simulink library "adc"  (Simulink 8.1)
settings: Solver=ode45  StartTime=0.0  StopTime=10.0  RelTol=1e-3
undefined symbols (not defined in the file or in its folder): KJUD_AEBDeactVehSpeed_mps, KJUD_AEBVehAssignTimer_ms
libraries: ava x1, hcu_lib x1
settings Model: Creator=xsellart  LastModifiedBy=tescamilla

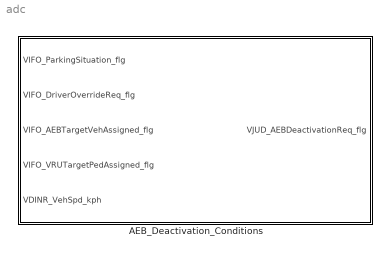
== system adc ==
  AEB_Deactivation_Conditions : Subsystem

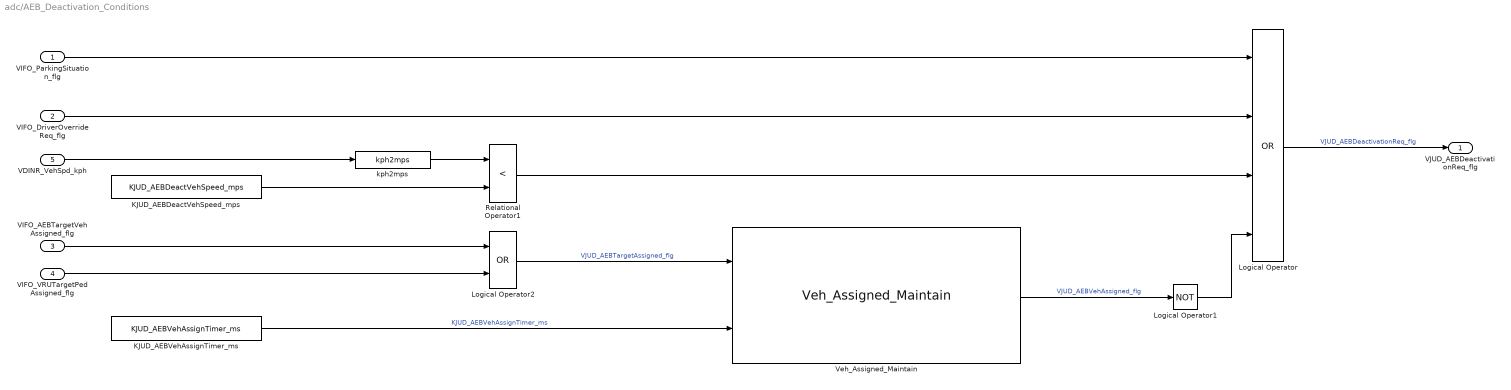
== system adc/AEB_Deactivation_Conditions ==
  VIFO_ParkingSituation_flg : Inport
  VIFO_DriverOverrideReq_flg : Inport  Port=2
  VIFO_AEBTargetVehAssigned_flg : Inport  Port=3
  VIFO_VRUTargetPedAssigned_flg : Inport  Port=4
  VDINR_VehSpd_kph : Inport  Port=5
  KJUD_AEBDeactVehSpeed_mps : Constant  Value=KJUD_AEBDeactVehSpeed_mps  OutDataTypeStr=single
  KJUD_AEBVehAssignTimer_ms : Constant  Value=KJUD_AEBVehAssignTimer_ms  OutDataTypeStr=single
  Logical Operator : Logic  Operator=OR  Inputs=4  AllPortsSameDT=off  OutDataTypeStr=boolean
  Logical Operator1 : Logic  Operator=NOT  AllPortsSameDT=off  OutDataTypeStr=boolean
  Logical Operator2 : Logic  Operator=OR  AllPortsSameDT=off  OutDataTypeStr=boolean
  Relational Operator1 : RelationalOperator  Operator=<  OutDataTypeStr=boolean
  Veh_Assigned_Maintain : ava/Veh_Assigned_Maintain
  kph2mps : hcu_lib/kph2mps
  VJUD_AEBDeactivationReq_flg : Outport
  wires:
  Logical Operator/1 -> VJUD_AEBDeactivationReq_flg/1  "VJUD_AEBDeactivationReq_flg"
  VIFO_AEBTargetVehAssigned_flg/1 -> Logical Operator2/1
  Relational Operator1/1 -> Logical Operator/3
  KJUD_AEBDeactVehSpeed_mps/1 -> Relational Operator1/2
  VDINR_VehSpd_kph/1 -> kph2mps/1
  VIFO_DriverOverrideReq_flg/1 -> Logical Operator/2
  VIFO_ParkingSituation_flg/1 -> Logical Operator/1
  Logical Operator1/1 -> Logical Operator/4
  KJUD_AEBVehAssignTimer_ms/1 -> Veh_Assigned_Maintain/2  "KJUD_AEBVehAssignTimer_ms"
  Veh_Assigned_Maintain/1 -> Logical Operator1/1  "VJUD_AEBVehAssigned_flg"
  kph2mps/1 -> Relational Operator1/1
  VIFO_VRUTargetPedAssigned_flg/1 -> Logical Operator2/2
  Logical Operator2/1 -> Veh_Assigned_Maintain/1  "VJUD_AEBTargetAssigned_flg"
